simulink model "lag"  (R2019a)
settings: Solver=VariableStepAuto  StartTime=0.0  StopTime=inf  RelTol=1e-3  EnableMultiTasking=on
undefined symbols (not defined in the file): f
libraries: instrumentlib x2
settings Model: Creator=Sony  LastModifiedBy=ilya
settings DataIOCC: LimitDataPoints=on  ReturnWorkspaceOutputs=off
settings OptimizationCC: LifeSpan=inf
settings DebuggingCC: AllowSymbolicDim=off  SFUnexpectedBacktrackingDiag=warning  SFNoUnconditionalDefaultTransitionDiag=warning  SFExecutionAtInitializationDiag=none  ArithmeticOperatorsInVariantConditions=warning
settings ModelReferenceCC: PropagateSignalLabelsOutOfModel=off
settings SFSimCC: SimUseLocalCustomCode=off
settings RTWCC: RTWUseLocalCustomCode=off
settings CodeAppCC: StateflowObjectComments=on
settings GRTTargetCC: TargetLangStandard=C89/C90 (ANSI)
settings ConfigComp: CovMetricSettings=dw  CovHtmlReporting=on  CovSaveCumulativeToWorkspaceVar=on  CovSaveSingleToWorkspaceVar=on  CovExternalEMLEnable=off

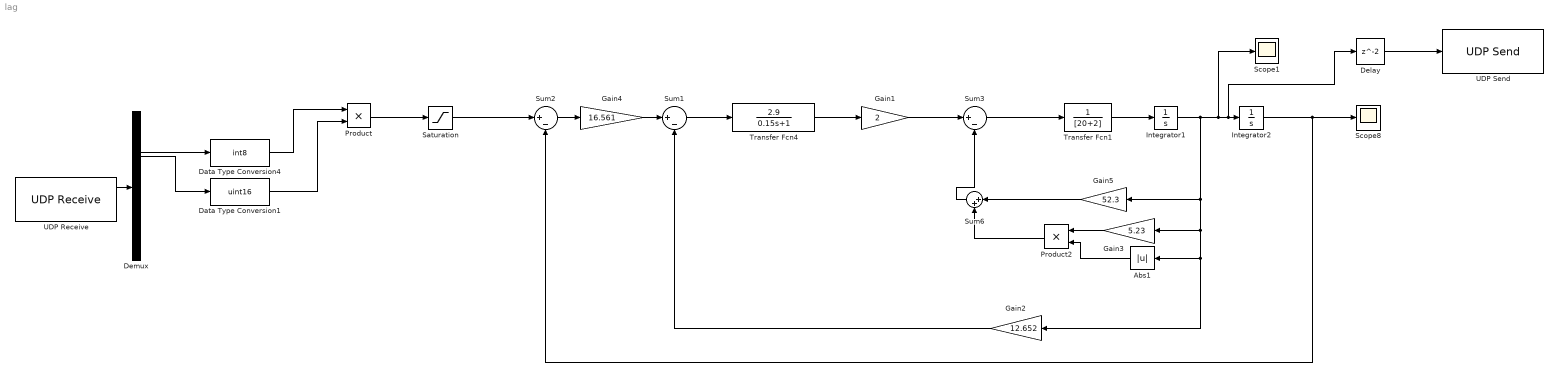
== system lag ==
  Abs1 : Abs
  Data Type Conversion1 : DataTypeConversion  OutMin=[1]  OutMax=1  OutDataTypeStr=uint16
  Data Type Conversion4 : DataTypeConversion  OutMin=[1]  OutMax=1  OutDataTypeStr=int8
  Delay : Delay
  Demux : Demux  Outputs=26
  Gain1 : Gain  Gain=2
  Gain2 : Gain  Gain=12.652
  Gain3 : Gain  Gain=5.23
  Gain4 : Gain  Gain=16.561
  Gain5 : Gain  Gain=52.3
  Integrator1 : Integrator
  Integrator2 : Integrator
  Product : Product
  Product2 : Product  RndMeth=Zero
  Saturation : Saturate  UpperLimit=3  LowerLimit=-3
  Scope1 : Scope
  Scope8 : Scope
  Sum1 : Sum  Inputs=|+-
  Sum2 : Sum  Inputs=|+-
  Sum3 : Sum  Inputs=|+-
  Sum6 : Sum  Inputs=|++
  Transfer Fcn1 : TransferFcn  Denominator=[20+2]
  Transfer Fcn4 : TransferFcn  Numerator=[2.9]  Denominator=[0.15 1]
  UDP Receive : instrumentlib/UDP Receive  Host=localhost  Port=9095  LocalPort=9095  EnablePortSharing=off  GetLatestData=off  DataSize="[26   1]"  DataType=uint8  ASCIIFormatting=%f,  Terminator=LF  ByteOrder=LittleEndian  EnableBlockingMode=off  Timeout=10  SampleTime=0.01  LocalAddress=127.0.0.1
      settings: SourceProductName=Instrument Control Toolbox
  UDP Send : instrumentlib/UDP Send  Host=127.0.0.1  Port=9090  LocalPort=-1  EnablePortSharing=off  ByteOrder=BigEndian  OutputDatagramPacketSize=512  EnableBlockingMode=off  LocalAddress=0.0.0.0
      settings: SourceProductName=Instrument Control Toolbox
  wires:
  Sum3/1 -> Transfer Fcn1/1
  Gain5/1 -> Sum6/1
  Transfer Fcn4/1 -> Gain1/1
  Sum6/1 -> Sum3/2
  Transfer Fcn1/1 -> Integrator1/1
  Gain1/1 -> Sum3/1
  Gain2/1 -> Sum1/2
  Integrator1/1 -> Scope1/1, Delay/1, Integrator2/1, Gain3/1, Abs1/1, Gain2/1, Gain5/1
  Sum2/1 -> Gain4/1
  Sum1/1 -> Transfer Fcn4/1
  Abs1/1 -> Product2/2
  Product2/1 -> Sum6/2
  Gain3/1 -> Product2/1
  Gain4/1 -> Sum1/1
  Integrator2/1 -> Sum2/2, Scope8/1
  Delay/1 -> UDP Send/1
  UDP Receive/1 -> Demux/1
  Demux/6 -> Data Type Conversion1/1
  Demux/5 -> Data Type Conversion4/1
  Data Type Conversion1/1 -> Product/2
  Data Type Conversion4/1 -> Product/1
  Product/1 -> Saturation/1
  Saturation/1 -> Sum2/1
